simulink model "opv_receiver_HDL_coder_input"  (R2023a)
settings: Solver=FixedStepDiscrete  StartTime=0.0  StopTime=0.01*(samples_per_frame/sample_rate)  RelTol=1e-3
values from neighbouring files (symbols this model uses):
  bits_per_symbol = 2    [opv.m]
  compFilt = design(compSpec,'SystemObject',true)    [opv.m]
  device_clock = 245.76e6    (= 245760000)    [opv.m]
  f1 = channel_center_frequency - outer_deviation    (= 57800)    [opv.m]
  f2 = channel_center_frequency - inner_deviation    (= 71350)    [opv.m]
  f3 = channel_center_frequency + inner_deviation    (= 84900)    [opv.m]
  f4 = channel_center_frequency + outer_deviation    (= 98450)    [opv.m]
  finalFilt = design(finalSpec,'equiripple','SystemObject',true)    [opv.m]
  symbol_rate = 27100    [opv.m]
undefined symbols (not defined in the file or in its folder): hbFilt, magnitude
libraries: dsphdlfiltering2 x32, dspsrcs4 x12, commrandsrc3 x8, dsphdlsigops2 x4
settings Model: Creator=matt  LastModifiedBy=matt
settings OptimizationCC: BlockReduction=off  ConditionallyExecuteInputs=off  DefaultParameterBehavior=Inlined
settings DebuggingCC: AlgebraicLoopMsg=error
settings HardwareCC: ProdBitPerPointer=32  ProdBitPerSizeT=32  ProdBitPerPtrDiffT=32  ProdLargestAtomicFloat=None  ProdIntDivRoundTo=Undefined  ProdEndianess=Unspecified  ProdWordSize=32  ProdHWDeviceType=ASIC/FPGA->ASIC/FPGA  TargetBitPerLong=64  TargetBitPerPointer=64  TargetBitPerSizeT=64  TargetBitPerPtrDiffT=64  TargetLongLongMode=on  TargetIntDivRoundTo=Zero  TargetEndianess=LittleEndian  TargetWordSize=64  TargetHWDeviceType=Custom Processor->MATLAB Host Computer  ProdEqTarget=off

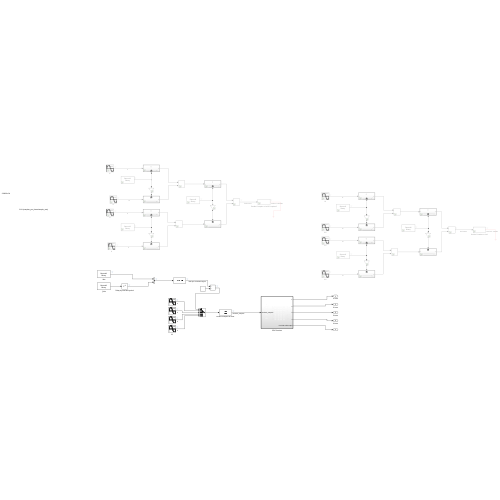
[thumbnail: Simulink's stored preview of the top-level diagram]
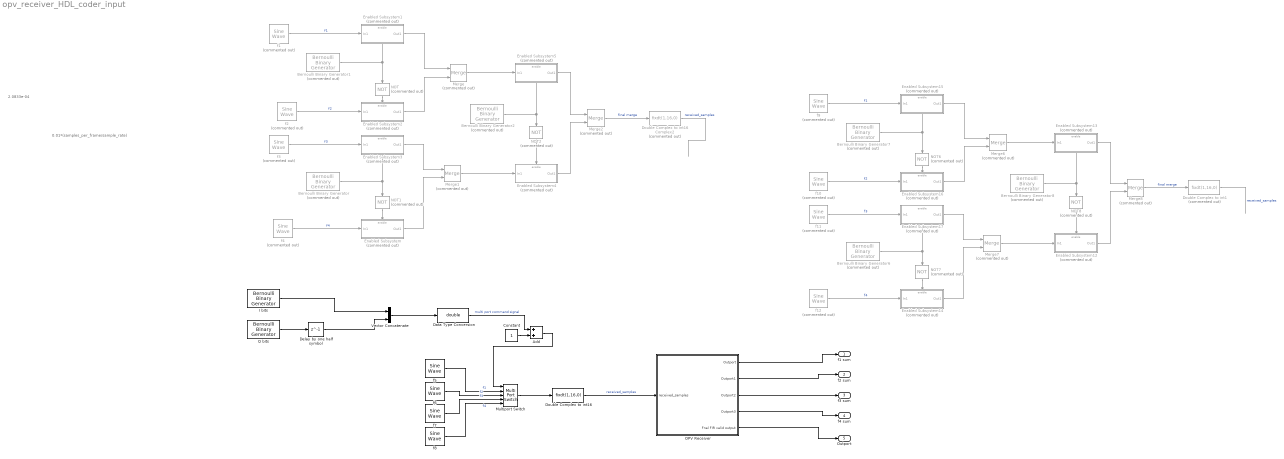
== system opv_receiver_HDL_coder_input ==
  note: 0.01*(samples_per_frame/sample_rate)
  note: 2.0833e-04
  Add : Sum
  Bernoulli Binary Generator{,1..2,6..8} (6 alike) : commrandsrc3/Bernoulli Binary Generator  Commented=on  ProbabilityOfZero=0.5  SeedSource=Auto  Seed=0  SampleTime=1/symbol_rate  SamplesPerFrame=1  OutputDataType=boolean  SimulateUsing=Interpreted execution
  Constant : Constant  SampleTime=1/(bits_per_symbol*symbol_rate)
  Data Type Conversion : DataTypeConversion  OutDataTypeStr=double  SaturateOnIntegerOverflow=off  RndMeth=Floor
  Delay by one half symbol : Delay  DelayLength=1  SampleTime=1/(bits_per_symbol*symbol_rate)
  Double Complex to int1 : DataTypeConversion  Commented=on  OutMin=[-32768]  OutMax=[32767]  OutDataTypeStr=fixdt(1,16,0)  ConvertRealWorld=Stored Integer (SI)  RndMeth=Floor
  Double Complex to int16 : DataTypeConversion  OutMin=[-32768]  OutMax=[32767]  OutDataTypeStr=fixdt(1,16,0)  ConvertRealWorld=Stored Integer (SI)  RndMeth=Floor
  Double Complex to int16 Complex2 : DataTypeConversion  Commented=on  OutMin=[-32768]  OutMax=[32767]  OutDataTypeStr=fixdt(1,16,0)  ConvertRealWorld=Stored Integer (SI)  RndMeth=Floor
  Enabled Subsystem : Subsystem  Commented=on  TreatAsAtomicUnit=on
      settings: LibrarySourceBlock=|
      | hdlsllib/Ports &
      | Subsystems/Enabled
      | Subsystem
  Enabled Subsystem1 : Subsystem  Commented=on  TreatAsAtomicUnit=on
      settings: LibrarySourceBlock=|
      | hdlsllib/Ports &
      | Subsystems/Enabled
      | Subsystem
  Enabled Subsystem12 : Subsystem  Commented=on  TreatAsAtomicUnit=on
      settings: LibrarySourceBlock=|
      | hdlsllib/Ports &
      | Subsystems/Enabled
      | Subsystem
  Enabled Subsystem13 : Subsystem  Commented=on  TreatAsAtomicUnit=on
      settings: LibrarySourceBlock=|
      | hdlsllib/Ports &
      | Subsystems/Enabled
      | Subsystem
  Enabled Subsystem14 : Subsystem  Commented=on  TreatAsAtomicUnit=on
      settings: LibrarySourceBlock=|
      | hdlsllib/Ports &
      | Subsystems/Enabled
      | Subsystem
  Enabled Subsystem15 : Subsystem  Commented=on  TreatAsAtomicUnit=on
      settings: LibrarySourceBlock=|
      | hdlsllib/Ports &
      | Subsystems/Enabled
      | Subsystem
  Enabled Subsystem16 : Subsystem  Commented=on  TreatAsAtomicUnit=on
      settings: LibrarySourceBlock=|
      | hdlsllib/Ports &
      | Subsystems/Enabled
      | Subsystem
  Enabled Subsystem17 : Subsystem  Commented=on  TreatAsAtomicUnit=on
      settings: LibrarySourceBlock=|
      | hdlsllib/Ports &
      | Subsystems/Enabled
      | Subsystem
  Enabled Subsystem2 : Subsystem  Commented=on  TreatAsAtomicUnit=on
      settings: LibrarySourceBlock=|
      | hdlsllib/Ports &
      | Subsystems/Enabled
      | Subsystem
  Enabled Subsystem3 : Subsystem  Commented=on  TreatAsAtomicUnit=on
      settings: LibrarySourceBlock=|
      | hdlsllib/Ports &
      | Subsystems/Enabled
      | Subsystem
  Enabled Subsystem4 : Subsystem  Commented=on  TreatAsAtomicUnit=on
      settings: LibrarySourceBlock=|
      | hdlsllib/Ports &
      | Subsystems/Enabled
      | Subsystem
  Enabled Subsystem5 : Subsystem  Commented=on  TreatAsAtomicUnit=on
      settings: LibrarySourceBlock=|
      | hdlsllib/Ports &
      | Subsystems/Enabled
      | Subsystem
  I bits : commrandsrc3/Bernoulli Binary Generator  ProbabilityOfZero=0.5  SeedSource=Auto  Seed=0  SampleTime=1/(symbol_rate)  SamplesPerFrame=1  OutputDataType=boolean  SimulateUsing=Interpreted execution
  Merge{,1..2,6..8} (6 alike) : Merge  Commented=on
  Multiport Switch : MultiPortSwitch  Inputs=4  DataPortIndices={1,2,3,4}  SaturateOnIntegerOverflow=off  InputSameDT=off
  NOT{,1..2,6..8} (6 alike) : Logic  Commented=on  Operator=NOT  IconShape=distinctive  AllPortsSameDT=off  OutDataTypeStr=boolean
  OPV Receiver : Subsystem  TreatAsAtomicUnit=on
      settings: LibrarySourceBlock=|
      | hdlsllib/Ports &
      | Subsystems/Subsystem
  Q bits : commrandsrc3/Bernoulli Binary Generator  ProbabilityOfZero=0.5  SeedSource=Auto  Seed=0  SampleTime=1/(symbol_rate)  SamplesPerFrame=1  OutputDataType=boolean  SimulateUsing=Interpreted execution
  Vector Concatenate : Concatenate
  f1 : dspsrcs4/Sine Wave  Commented=on  Amplitude=2^15-1  Frequency=f1  Phase=0  SampleMode=Discrete  OutComplex=Complex  CompMethod=Trigonometric fcn  TableSize=Speed  SampleTime=1/device_clock  SamplesPerFrame=1  ResetState=Restart at time zero  OutputFrames=off  dataType=double  wordLen=16  udDataType=sfix(16)  fracBitsMode=User-defined  numFracBits=0  OutDataTypeStr=double  LastOutDataTypeStr=double
  f10 : dspsrcs4/Sine Wave  Commented=on  Amplitude=2^15-1  Frequency=f2  Phase=0  SampleMode=Discrete  OutComplex=Real  CompMethod=Trigonometric fcn  TableSize=Speed  SampleTime=1/device_clock  SamplesPerFrame=1  ResetState=Restart at time zero  OutputFrames=off  dataType=double  wordLen=16  udDataType=sfix(16)  fracBitsMode=User-defined  numFracBits=0  OutDataTypeStr=double  LastOutDataTypeStr=double
  f11 : dspsrcs4/Sine Wave  Commented=on  Amplitude=2^15-1  Frequency=f3  Phase=0  SampleMode=Discrete  OutComplex=Real  CompMethod=Trigonometric fcn  TableSize=Speed  SampleTime=1/device_clock  SamplesPerFrame=1  ResetState=Restart at time zero  OutputFrames=off  dataType=double  wordLen=16  udDataType=sfix(16)  fracBitsMode=User-defined  numFracBits=0  OutDataTypeStr=double  LastOutDataTypeStr=double
  f12 : dspsrcs4/Sine Wave  Commented=on  Amplitude=2^15-1  Frequency=f4  Phase=0  SampleMode=Discrete  OutComplex=Real  CompMethod=Trigonometric fcn  TableSize=Speed  SampleTime=1/device_clock  SamplesPerFrame=1  ResetState=Restart at time zero  OutputFrames=off  dataType=double  wordLen=16  udDataType=sfix(16)  fracBitsMode=User-defined  numFracBits=0  OutDataTypeStr=double  LastOutDataTypeStr=double
  f2 : dspsrcs4/Sine Wave  Commented=on  Amplitude=2^15-1  Frequency=f2  Phase=0  SampleMode=Discrete  OutComplex=Complex  CompMethod=Trigonometric fcn  TableSize=Speed  SampleTime=1/device_clock  SamplesPerFrame=1  ResetState=Restart at time zero  OutputFrames=off  dataType=double  wordLen=16  udDataType=sfix(16)  fracBitsMode=User-defined  numFracBits=0  OutDataTypeStr=double  LastOutDataTypeStr=double
  f3 : dspsrcs4/Sine Wave  Commented=on  Amplitude=2^15-1  Frequency=f3  Phase=0  SampleMode=Discrete  OutComplex=Complex  CompMethod=Trigonometric fcn  TableSize=Speed  SampleTime=1/device_clock  SamplesPerFrame=1  ResetState=Restart at time zero  OutputFrames=off  dataType=double  wordLen=16  udDataType=sfix(16)  fracBitsMode=User-defined  numFracBits=0  OutDataTypeStr=double  LastOutDataTypeStr=double
  f4 : dspsrcs4/Sine Wave  Commented=on  Amplitude=2^15-1  Frequency=f4  Phase=0  SampleMode=Discrete  OutComplex=Complex  CompMethod=Trigonometric fcn  TableSize=Speed  SampleTime=1/device_clock  SamplesPerFrame=1  ResetState=Restart at time zero  OutputFrames=off  dataType=double  wordLen=16  udDataType=sfix(16)  fracBitsMode=User-defined  numFracBits=0  OutDataTypeStr=double  LastOutDataTypeStr=double
  f5 : dspsrcs4/Sine Wave  Amplitude=2^15-1  Frequency=f1  Phase=0  SampleMode=Discrete  OutComplex=Real  CompMethod=Trigonometric fcn  TableSize=Speed  SampleTime=1/device_clock  SamplesPerFrame=1  ResetState=Restart at time zero  OutputFrames=off  dataType=double  wordLen=16  udDataType=sfix(16)  fracBitsMode=User-defined  numFracBits=0  OutDataTypeStr=double  LastOutDataTypeStr=double
  f6 : dspsrcs4/Sine Wave  Amplitude=2^15-1  Frequency=f2  Phase=0  SampleMode=Discrete  OutComplex=Real  CompMethod=Trigonometric fcn  TableSize=Speed  SampleTime=1/device_clock  SamplesPerFrame=1  ResetState=Restart at time zero  OutputFrames=off  dataType=double  wordLen=16  udDataType=sfix(16)  fracBitsMode=User-defined  numFracBits=0  OutDataTypeStr=double  LastOutDataTypeStr=double
  f7 : dspsrcs4/Sine Wave  Amplitude=2^15-1  Frequency=f3  Phase=0  SampleMode=Discrete  OutComplex=Real  CompMethod=Trigonometric fcn  TableSize=Speed  SampleTime=1/device_clock  SamplesPerFrame=1  ResetState=Restart at time zero  OutputFrames=off  dataType=double  wordLen=16  udDataType=sfix(16)  fracBitsMode=User-defined  numFracBits=0  OutDataTypeStr=double  LastOutDataTypeStr=double
  f8 : dspsrcs4/Sine Wave  Amplitude=2^15-1  Frequency=f4  Phase=0  SampleMode=Discrete  OutComplex=Real  CompMethod=Trigonometric fcn  TableSize=Speed  SampleTime=1/device_clock  SamplesPerFrame=1  ResetState=Restart at time zero  OutputFrames=off  dataType=double  wordLen=16  udDataType=sfix(16)  fracBitsMode=User-defined  numFracBits=0  OutDataTypeStr=double  LastOutDataTypeStr=double
  f9 : dspsrcs4/Sine Wave  Commented=on  Amplitude=2^15-1  Frequency=f1  Phase=0  SampleMode=Discrete  OutComplex=Real  CompMethod=Trigonometric fcn  TableSize=Speed  SampleTime=1/device_clock  SamplesPerFrame=1  ResetState=Restart at time zero  OutputFrames=off  dataType=double  wordLen=16  udDataType=sfix(16)  fracBitsMode=User-defined  numFracBits=0  OutDataTypeStr=double  LastOutDataTypeStr=double
  f1 sum : Outport
  f2 sum : Outport  Port=2
  f3 sum : Outport  Port=3
  f4 sum : Outport  Port=4
  Outport : Outport  Port=5
  wires:
  Enabled Subsystem1/1(Out1) -> Merge/1
  Bernoulli Binary Generator1/1 -> NOT/1, Enabled Subsystem1/Enable
  NOT/1 -> Enabled Subsystem2/Enable
  Enabled Subsystem2/1(Out1) -> Merge/2
  NOT1/1 -> Enabled Subsystem/Enable
  Bernoulli Binary Generator/1 -> NOT1/1, Enabled Subsystem3/Enable
  Enabled Subsystem3/1(Out1) -> Merge1/1
  Enabled Subsystem/1(Out1) -> Merge1/2
  NOT2/1 -> Enabled Subsystem4/Enable
  Bernoulli Binary Generator2/1 -> NOT2/1, Enabled Subsystem5/Enable
  Merge1/1 -> Enabled Subsystem4/1(In1)
  Merge/1 -> Enabled Subsystem5/1(In1)
  Enabled Subsystem5/1(Out1) -> Merge2/1
  Enabled Subsystem4/1(Out1) -> Merge2/2
  Merge2/1 -> Double Complex to int16 Complex2/1  "final merge"
  Double Complex to int16 Complex2/1 -> ?  "received_samples"
  f1/1 -> Enabled Subsystem1/1(In1)  "f1"
  f2/1 -> Enabled Subsystem2/1(In1)  "f2"
  f3/1 -> Enabled Subsystem3/1(In1)  "f3"
  f4/1 -> Enabled Subsystem/1(In1)  "f4"
  OPV Receiver/2(Outport1) -> f2 sum/1
  OPV Receiver/1(Outport) -> f1 sum/1
  OPV Receiver/4(Outport3) -> f4 sum/1
  OPV Receiver/3(Outport2) -> f3 sum/1
  OPV Receiver/5(Fnal FIR valid output) -> Outport/1
  Double Complex to int16/1 -> OPV Receiver/1(received_samples)  "received_samples"
  Enabled Subsystem14/1(Out1) -> Merge7/2
  Merge7/1 -> Enabled Subsystem12/1(In1)
  NOT8/1 -> Enabled Subsystem12/Enable
  Merge6/1 -> Enabled Subsystem13/1(In1)
  Enabled Subsystem12/1(Out1) -> Merge8/2
  Bernoulli Binary Generator6/1 -> NOT7/1, Enabled Subsystem17/Enable
  NOT6/1 -> Enabled Subsystem16/Enable
  f12/1 -> Enabled Subsystem14/1(In1)  "f4"
  Bernoulli Binary Generator8/1 -> NOT8/1, Enabled Subsystem13/Enable
  Enabled Subsystem17/1(Out1) -> Merge7/1
  Enabled Subsystem16/1(Out1) -> Merge6/2
  Double Complex to int1/1 -> ?  "received_samples"
  Bernoulli Binary Generator7/1 -> NOT6/1, Enabled Subsystem15/Enable
  NOT7/1 -> Enabled Subsystem14/Enable
  Enabled Subsystem15/1(Out1) -> Merge6/1
  Merge8/1 -> Double Complex to int1/1  "final merge"
  f11/1 -> Enabled Subsystem17/1(In1)  "f3"
  f10/1 -> Enabled Subsystem16/1(In1)  "f2"
  Enabled Subsystem13/1(Out1) -> Merge8/1
  f9/1 -> Enabled Subsystem15/1(In1)  "f1"
  Q bits/1 -> Delay by one half symbol/1
  I bits/1 -> Vector Concatenate/1
  Delay by one half symbol/1 -> Vector Concatenate/2
  Vector Concatenate/1 -> Data Type Conversion/1
  Multiport Switch/1 -> Double Complex to int16/1
  Data Type Conversion/1 -> Add/1  "multi port command signal"
  f7/1 -> Multiport Switch/4  "f3"
  f8/1 -> Multiport Switch/5  "f4"
  f6/1 -> Multiport Switch/3  "f2"
  f5/1 -> Multiport Switch/2  "f1"
  Constant/1 -> Add/2
  Add/1 -> Multiport Switch/1

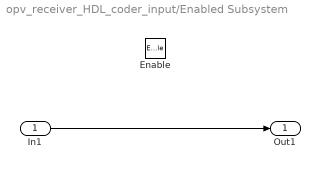
== system opv_receiver_HDL_coder_input/Enabled Subsystem ==
  In1 : Inport
  Enable : EnablePort
  Out1 : Outport
  wires:
  In1/1 -> Out1/1

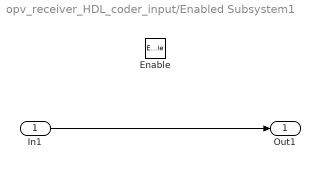
== system opv_receiver_HDL_coder_input/Enabled Subsystem1 ==
  In1 : Inport
  Enable : EnablePort
  Out1 : Outport
  wires:
  In1/1 -> Out1/1

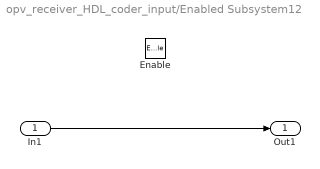
== system opv_receiver_HDL_coder_input/Enabled Subsystem12 ==
  In1 : Inport
  Enable : EnablePort
  Out1 : Outport
  wires:
  In1/1 -> Out1/1

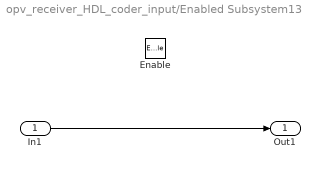
== system opv_receiver_HDL_coder_input/Enabled Subsystem13 ==
  In1 : Inport
  Enable : EnablePort
  Out1 : Outport
  wires:
  In1/1 -> Out1/1

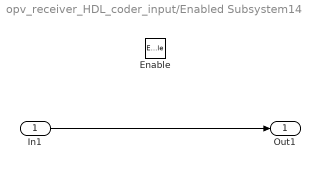
== system opv_receiver_HDL_coder_input/Enabled Subsystem14 ==
  In1 : Inport
  Enable : EnablePort
  Out1 : Outport
  wires:
  In1/1 -> Out1/1

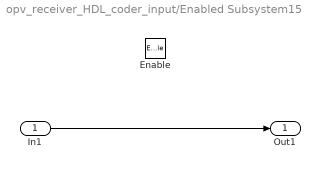
== system opv_receiver_HDL_coder_input/Enabled Subsystem15 ==
  In1 : Inport
  Enable : EnablePort
  Out1 : Outport
  wires:
  In1/1 -> Out1/1

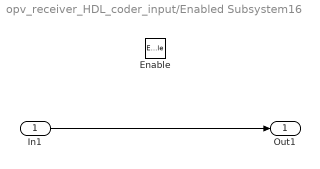
== system opv_receiver_HDL_coder_input/Enabled Subsystem16 ==
  In1 : Inport
  Enable : EnablePort
  Out1 : Outport
  wires:
  In1/1 -> Out1/1

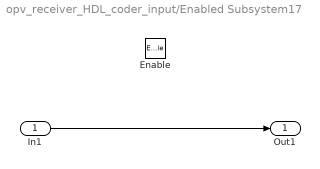
== system opv_receiver_HDL_coder_input/Enabled Subsystem17 ==
  In1 : Inport
  Enable : EnablePort
  Out1 : Outport
  wires:
  In1/1 -> Out1/1

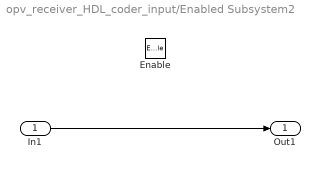
== system opv_receiver_HDL_coder_input/Enabled Subsystem2 ==
  In1 : Inport
  Enable : EnablePort
  Out1 : Outport
  wires:
  In1/1 -> Out1/1

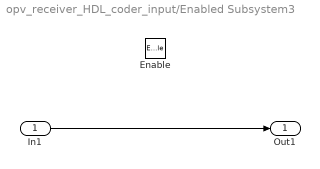
== system opv_receiver_HDL_coder_input/Enabled Subsystem3 ==
  In1 : Inport
  Enable : EnablePort
  Out1 : Outport
  wires:
  In1/1 -> Out1/1

== system opv_receiver_HDL_coder_input/Enabled Subsystem4 ==
  In1 : Inport
  Enable : EnablePort
  Out1 : Outport
  wires:
  In1/1 -> Out1/1

== system opv_receiver_HDL_coder_input/Enabled Subsystem5 ==
  In1 : Inport
  Enable : EnablePort
  Out1 : Outport
  wires:
  In1/1 -> Out1/1

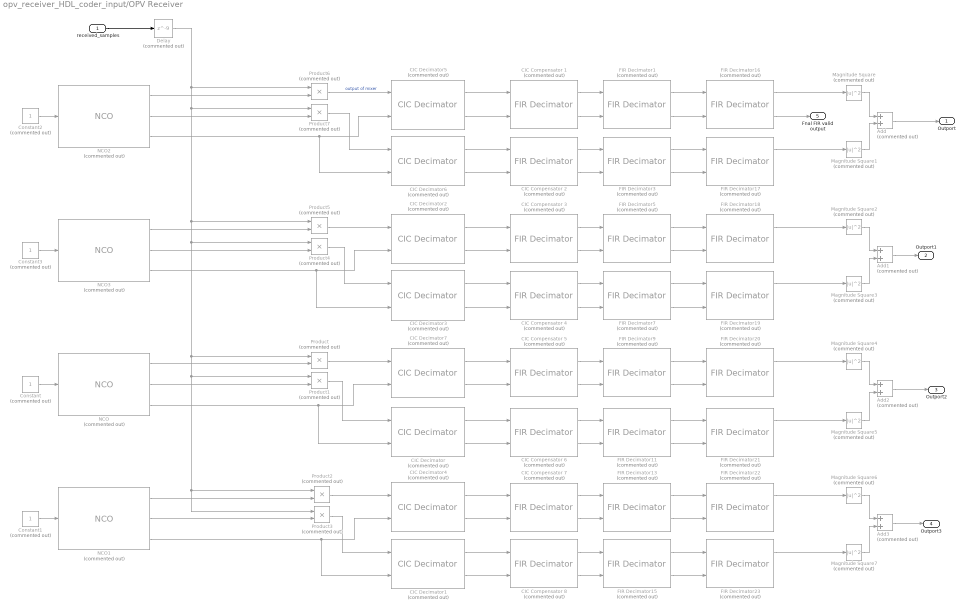
== system opv_receiver_HDL_coder_input/OPV Receiver ==
  received_samples : Inport
  Add{,1..3} (4 alike) : Sum  Commented=on
  CIC Compensator {1..8} (8 alike) : dsphdlfiltering2/FIR Decimator  Commented=on  Numerator=compFilt.Numerator  FilterStructure=Direct form systolic  DecimationFactor=2  NumCycles=2  SimulateUsing=Code generation  roundingMode=Floor  overflowMode=off  CoefficientsDataTypeStr=Inherit: Same word length as input  OutputDataTypeStr=fixdt(1,16,0)  ResetInputPort=off  HDLGlobalReset=off
  CIC Decimator{,1..7} (8 alike) : dsphdlfiltering2/CIC Decimator  Commented=on  DecimationSource=Property  DecimationFactor=cicParams.DecimationFactor  MaxDecimationFactor=2  DifferentialDelay=cicParams.DifferentialDelay  NumSections=cicParams.NumSections  GainCorrection=on  SimulateUsing=Code generation  OutputDataType=Minimum section word lengths  OutputWordLength=16  ResetInputPort=off  HDLGlobalReset=off
  Constant{,1..3} (4 alike) : Constant  Commented=on  OutDataTypeStr=boolean  SampleTime=1/(device_clock)
  Delay : Delay  Commented=on  DelayLength=9  InitialCondition=0
  FIR Decimator{1,3,5,7,9,11,13,15} (8 alike) : dsphdlfiltering2/FIR Decimator  Commented=on  Numerator=hbFilt.Numerator  FilterStructure=Direct form systolic  DecimationFactor=2  NumCycles=4  SimulateUsing=Code generation  roundingMode=Floor  overflowMode=off  CoefficientsDataTypeStr=Inherit: Same word length as input  OutputDataTypeStr=fixdt(1,16,0)  ResetInputPort=off  HDLGlobalReset=off
  FIR Decimator{16..23} (8 alike) : dsphdlfiltering2/FIR Decimator  Commented=on  Numerator=finalFilt.Numerator  FilterStructure=Direct form systolic  DecimationFactor=2  NumCycles=8  SimulateUsing=Code generation  roundingMode=Floor  overflowMode=off  CoefficientsDataTypeStr=Inherit: Same word length as input  OutputDataTypeStr=fixdt(1,16,0)  ResetInputPort=off  HDLGlobalReset=off
  Magnitude Square{,1..7} (8 alike) : Math  Commented=on  Operator=magnitude^2  SignedPower=on  RndMeth=Zero  OutDataTypeStr=Inherit: Inherit via internal rule
  NCO : dsphdlsigops2/NCO  Commented=on  PhaseIncrementSource=Property  PhaseIncrement=phase_increment_f3  PhaseOffsetSource=Property  PhaseOffset=0  DitherSource=Property  NumDitherBits=16  SamplesPerFrame=1  LUTCompress=off  ResetAction=off  Waveform=Sine and cosine  PhasePort=off  SimulateUsing=Code generation  AccumulatorWL=32  PhaseQuantization=on  NumQuantizerAccumulatorBits=12  OutputDataType=Binary point scaling  OutputWL=16  OutputFL=14
      settings: LibrarySourceBlock=dsphdlsrcs2/NCO
  NCO1 : dsphdlsigops2/NCO  Commented=on  PhaseIncrementSource=Property  PhaseIncrement=phase_increment_f4  PhaseOffsetSource=Property  PhaseOffset=0  DitherSource=Property  NumDitherBits=16  SamplesPerFrame=1  LUTCompress=off  ResetAction=off  Waveform=Sine and cosine  PhasePort=off  SimulateUsing=Code generation  AccumulatorWL=32  PhaseQuantization=on  NumQuantizerAccumulatorBits=12  OutputDataType=Binary point scaling  OutputWL=16  OutputFL=14
      settings: LibrarySourceBlock=dsphdlsrcs2/NCO
  NCO2 : dsphdlsigops2/NCO  Commented=on  PhaseIncrementSource=Property  PhaseIncrement=phase_increment_f1  PhaseOffsetSource=Property  PhaseOffset=0  DitherSource=Property  NumDitherBits=16  SamplesPerFrame=1  LUTCompress=off  ResetAction=off  Waveform=Sine and cosine  PhasePort=off  SimulateUsing=Code generation  AccumulatorWL=32  PhaseQuantization=on  NumQuantizerAccumulatorBits=12  OutputDataType=Binary point scaling  OutputWL=16  OutputFL=14
      settings: LibrarySourceBlock=dsphdlsrcs2/NCO
  NCO3 : dsphdlsigops2/NCO  Commented=on  PhaseIncrementSource=Property  PhaseIncrement=phase_increment_f2  PhaseOffsetSource=Property  PhaseOffset=0  DitherSource=Property  NumDitherBits=16  SamplesPerFrame=1  LUTCompress=off  ResetAction=off  Waveform=Sine and cosine  PhasePort=off  SimulateUsing=Code generation  AccumulatorWL=32  PhaseQuantization=on  NumQuantizerAccumulatorBits=12  OutputDataType=Binary point scaling  OutputWL=16  OutputFL=14
      settings: LibrarySourceBlock=dsphdlsrcs2/NCO
  Product{,1..7} (8 alike) : Product  Commented=on
  Outport : Outport
  Outport1 : Outport  Port=2
  Outport2 : Outport  Port=3
  Outport3 : Outport  Port=4
  Fnal FIR valid output : Outport  Port=5
  wires:
  Product1/1 -> CIC Decimator/1
  Product5/1 -> CIC Decimator2/1
  Product3/1 -> CIC Decimator1/1
  NCO1/3 -> CIC Decimator4/2, CIC Decimator1/2
  NCO1/2 -> Product3/2
  NCO/3 -> CIC Decimator7/2, CIC Decimator/2
  Product6/1 -> CIC Decimator5/1  "output of mixer"
  Constant2/1 -> NCO2/1
  Constant3/1 -> NCO3/1
  Product7/1 -> CIC Decimator6/1
  received_samples/1 -> Delay/1
  NCO2/3 -> CIC Decimator5/2, CIC Decimator6/2
  NCO1/1 -> Product2/2
  NCO/1 -> Product/2
  Constant/1 -> NCO/1
  Product4/1 -> CIC Decimator3/1
  Constant1/1 -> NCO1/1
  NCO2/1 -> Product6/2
  NCO2/2 -> Product7/2
  Product2/1 -> CIC Decimator4/1
  NCO3/1 -> Product5/2
  NCO3/2 -> Product4/2
  Product/1 -> CIC Decimator7/1
  NCO3/3 -> CIC Decimator3/2, CIC Decimator2/2
  NCO/2 -> Product1/2
  Delay/1 -> Product6/1, Product7/1, Product5/1, Product4/1, Product/1, Product1/1, Product2/1, Product3/1
  CIC Decimator5/1 -> CIC Compensator 1/1
  CIC Decimator6/1 -> CIC Compensator 2/1
  CIC Decimator5/2 -> CIC Compensator 1/2
  CIC Compensator 1/1 -> FIR Decimator1/1
  CIC Compensator 1/2 -> FIR Decimator1/2
  CIC Compensator 2/1 -> FIR Decimator3/1
  CIC Compensator 2/2 -> FIR Decimator3/2
  CIC Decimator6/2 -> CIC Compensator 2/2
  CIC Compensator 3/1 -> FIR Decimator5/1
  CIC Compensator 3/2 -> FIR Decimator5/2
  CIC Decimator2/1 -> CIC Compensator 3/1
  CIC Decimator2/2 -> CIC Compensator 3/2
  CIC Compensator 4/1 -> FIR Decimator7/1
  CIC Compensator 4/2 -> FIR Decimator7/2
  CIC Decimator3/1 -> CIC Compensator 4/1
  CIC Decimator3/2 -> CIC Compensator 4/2
  CIC Compensator 5/1 -> FIR Decimator9/1
  CIC Compensator 5/2 -> FIR Decimator9/2
  CIC Decimator7/1 -> CIC Compensator 5/1
  CIC Decimator7/2 -> CIC Compensator 5/2
  CIC Compensator 6/1 -> FIR Decimator11/1
  CIC Compensator 6/2 -> FIR Decimator11/2
  CIC Decimator/1 -> CIC Compensator 6/1
  CIC Decimator/2 -> CIC Compensator 6/2
  CIC Compensator 7/1 -> FIR Decimator13/1
  CIC Compensator 7/2 -> FIR Decimator13/2
  CIC Decimator4/1 -> CIC Compensator 7/1
  CIC Decimator4/2 -> CIC Compensator 7/2
  CIC Compensator 8/1 -> FIR Decimator15/1
  CIC Compensator 8/2 -> FIR Decimator15/2
  CIC Decimator1/1 -> CIC Compensator 8/1
  CIC Decimator1/2 -> CIC Compensator 8/2
  FIR Decimator1/1 -> FIR Decimator16/1
  FIR Decimator1/2 -> FIR Decimator16/2
  FIR Decimator3/2 -> FIR Decimator17/2
  FIR Decimator3/1 -> FIR Decimator17/1
  FIR Decimator5/2 -> FIR Decimator18/2
  FIR Decimator5/1 -> FIR Decimator18/1
  FIR Decimator7/2 -> FIR Decimator19/2
  FIR Decimator7/1 -> FIR Decimator19/1
  FIR Decimator9/2 -> FIR Decimator20/2
  FIR Decimator9/1 -> FIR Decimator20/1
  FIR Decimator11/2 -> FIR Decimator21/2
  FIR Decimator11/1 -> FIR Decimator21/1
  FIR Decimator13/2 -> FIR Decimator22/2
  FIR Decimator13/1 -> FIR Decimator22/1
  FIR Decimator15/2 -> FIR Decimator23/2
  FIR Decimator15/1 -> FIR Decimator23/1
  FIR Decimator16/1 -> Magnitude Square/1
  FIR Decimator17/1 -> Magnitude Square1/1
  FIR Decimator18/1 -> Magnitude Square2/1
  FIR Decimator19/1 -> Magnitude Square3/1
  FIR Decimator20/1 -> Magnitude Square4/1
  FIR Decimator21/1 -> Magnitude Square5/1
  FIR Decimator22/1 -> Magnitude Square6/1
  FIR Decimator23/1 -> Magnitude Square7/1
  Magnitude Square/1 -> Add/1
  Magnitude Square1/1 -> Add/2
  Magnitude Square3/1 -> Add1/2
  Magnitude Square2/1 -> Add1/1
  Magnitude Square4/1 -> Add2/1
  Magnitude Square5/1 -> Add2/2
  Magnitude Square7/1 -> Add3/2
  Magnitude Square6/1 -> Add3/1
  Add3/1 -> Outport3/1
  Add2/1 -> Outport2/1
  Add1/1 -> Outport1/1
  Add/1 -> Outport/1
  FIR Decimator16/2 -> Fnal FIR valid output/1
